simulink model "Offline_MiL_Sim_Public"  (R2024a)
settings: Solver=ode1  StartTime=0.0  StopTime=inf  FixedStep=step_size  RelTol=1e-3  EnableMultiTasking=on
PostLoadFcn:
  | if any(exist('dsrtsu_mdlpostloadfcn', 'file') ~= 0), dsrtsu_mdlpostloadfcn('Execute', bdroot); end
InitFcn:
  | , if any(exist('rtifpga_mdlclblib', 'file') ~= 0), rtifpga_mdlclblib('Init', bdroot); end,
  | , if any(exist('dsmpb_private', 'file') ~= 0), dsmpb_private('dsmpb_mdlclblib', 'Init', bdroot); end,
undefined symbols (not defined in the file or in its folder): Af, break_criteria, C_r, C_w, Cd, CurrentLosses, dens, DiscIntNeverNeededParam, FDR, fr, Friction, gain_Twr, grade_track, grav, IronLosses, Kp_c, lbh_ac, lbx_ac, lbx_ac_e, lbx_mhe, M_EM_acc_0, M_EM_acc_max, M_EM_brk_min, M_gen_max, M_mot_max, mpc_init_EM_acc, mpc_init_EM_brk, mpc_init_fric_brk, mps_kmh, Mv, n_0, n_em_max, n_gen_max, n_mot_max, n_vec, nout, numHiddenUnits, options, options_mhe, optparam, P, parameter_0, Q, R, r_dyn, R_w_c, R_w_e, R_w_r, rps_rpm, s_track, SE_selector_sim, start_distance_check, step_size, T_c, T_cool, T_e, T_init, T_max, t_mpc_on, T_r_0 ... (+21)
libraries: simulink x3, matrix_library x2, deeplib x1
(part 1 of 2)
PreSaveFcn:
  | if any(exist('dsmpb_private', 'file') ~= 0), dsmpb_private('dsmpb_mdlclblib', 'PreSave', bdroot); end
CloseFcn:
  | if any(exist('dsmpb_private', 'file') ~= 0), dsmpb_private('dsmpb_mdlclblib', 'Close', bdroot); end
settings Model: FPTRunName=Active  DSMPB_ID_DATA={}  RTICANMMDATA=struct('GeneralSetupData',struct('modelroot','D:\Git_Winkler\nmpc_wang','generalsettings',struct('filesettings',struct('destfolder',struct('Name','RTICANMM_FILES','Check',1),'buildfolder',struct('Name','.','Check',1),'AbsDestfolder',struct('Name','D:\Git_Winkler\nmpc_wang\RTICANMM_FILES'),'AbsBuildfolder',struct('Name','D:\Git_Winkler\nmpc_wang'))),'options',struct('addpaths',1,'rmpaths',1,'addtrcexclusion',true,'cannavigator',struct('checkmonitoring',0),'show_usrtrc',0,'use_usrtrc',0),'advanced',struct('options',ones(1,100)),'MPSetup',{{}},'RTI',struct('Type','DSRT','Ver','4.6','Date','02-Nov-2021'),'modelname','mpc_ww_Scalexio_Offline_LSTM_v3_2021a','block','mpc_ww_Scalexio_Offline_LSTM_v3_2021a'))  DSRTSU_INTERNAL_RTIFPGA=170  DSRTSU_INTERNAL_RTISTBM_VER=1.4.3  NumberOfSteps=10  PacingRate=1.600000  Creator=The MathWorks, Inc.  LastModifiedBy=winkler_a
settings SolverCC: AlgebraicLoopSolver=LineSearch  AutoInsertRateTranBlk=on
settings DataIOCC: SaveFormat=Array  SignalLogging=off  DSMLogging=off  ReturnWorkspaceOutputs=off  SignalLoggingName=sigsOut
settings OptimizationCC: BlockReduction=off  BooleanDataType=off  ConditionallyExecuteInputs=off  DefaultParameterBehavior=Inlined  OptimizeBlockIOStorage=off  BufferReuse=off  ReuseModelBlockBuffer=off  GlobalBufferReuse=off  ExpressionFolding=off  ExpressionDepthLimit=2147483647  LocalBlockOutputs=off  InitFltsAndDblsToZero=on  OptimizeDataStoreBuffers=off  BusAssignmentInplaceUpdate=off
settings DebuggingCC: SaveWithParameterizedLinksMsg=none  MultiTaskDSMMsg=warning  MultiTaskCondExecSysMsg=none  TasksWithSamePriorityMsg=none  FcnCallInpInsideContextMsg=warning  UnconnectedLineMsg=warning  StateNameClashWarn=warning  SFUnexpectedBacktrackingDiag=warning  SFNoUnconditionalDefaultTransitionDiag=warning  ArithmeticOperatorsInVariantConditions=warning
settings HardwareCC: ProdBitPerPointer=32  ProdBitPerSizeT=32  ProdBitPerPtrDiffT=32  ProdLargestAtomicInteger=Integer  ProdWordSize=32  ProdHWDeviceType=Custom Processor->Custom  TargetBitPerPointer=64  TargetBitPerSizeT=64  TargetBitPerPtrDiffT=64  TargetLongLongMode=on  TargetIntDivRoundTo=Zero  TargetEndianess=LittleEndian  TargetWordSize=64  TargetHWDeviceType=MATLAB Host
settings ModelReferenceCC: EnableRefExpFcnMdlSchedulingChecks=on  PropagateSignalLabelsOutOfModel=off
settings SFSimCC: SimUseLocalCustomCode=off  MATLABDynamicMemAlloc=off  CustomCodeUndefinedFunction=UseInterfaceOnly
settings RTWCC: Description=dSPACE Run-Time Target (for VEOS and ConfigurationDesk)  SystemTargetFile=dsrt.tlc  GenCodeOnly=on  MakeCommand=make_dsrt  TemplateMakefile=dsrt_default_tmf  RTWVerbose=off  RTWUseLocalCustomCode=off  GPUComputeCapability=3.5  DLArmComputeVersion=19.05
settings CodeAppCC: StateflowObjectComments=on
settings STFCustomTargetCC: TargetLangStandard=C89/C90 (ANSI)  ParMdlRefBuildCompliant=on  GRTInterface=off  UseToolchainInfoCompliant=off  SystemTargetFile=dsrt.tlc
settings GRTTargetCC: TargetLangStandard=C89/C90 (ANSI)  CompOptLevelCompliant=off  ConcurrentExecutionCompliant=off  CombineOutputUpdateFcns=off  MatFileLogging=off  CPPClassGenCompliant=off  UseToolchainInfoCompliant=off
settings ConfigComp: CovMetricSettings=dw  CovSaveCumulativeToWorkspaceVar=on  CovSaveSingleToWorkspaceVar=on  CovExternalEMLEnable=off  CovSFcnEnable=off

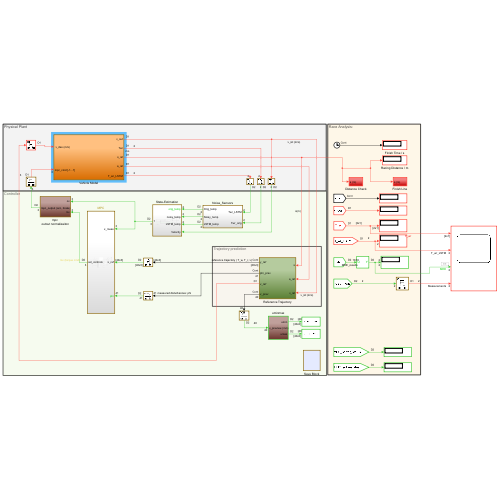
[thumbnail: Simulink's stored preview of the top-level diagram]
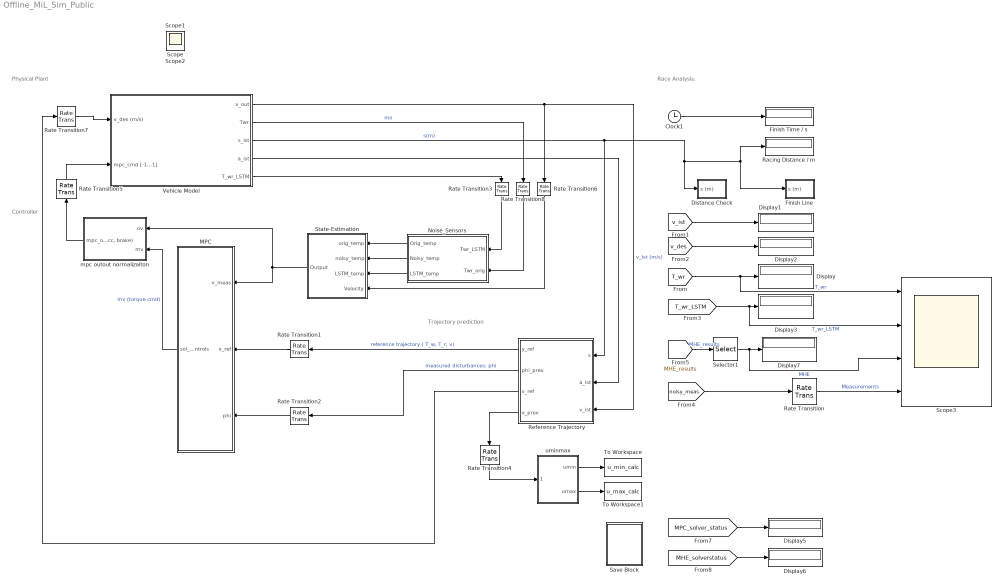
== system Offline_MiL_Sim_Public ==
  note: Trajectory prediction
  note: Controller
  note: Physical Plant
  note: Race Analysis:
  Clock1 : Clock
  Display{,1..3,5..7} (7 alike) : Display
  Distance Check : Subsystem
  Finish Line : Subsystem
  Finish Time / s : Display
  MPC : Subsystem
  Noise_Sensors : Subsystem
  Racing Distance / m : Display
  Rate Transition : RateTransition
  Rate Transition1 : RateTransition  InitialCondition=X0_ref  OutPortSampleTime=options.Ts
  Rate Transition2 : RateTransition  InitialCondition=parameter_0(1:(options.P+1))  OutPortSampleTime=options.Ts
  Rate Transition3 : RateTransition  Deterministic=off  InitialCondition=[T_w_0, T_r_0]  OutPortSampleTime=options.Ts
  Rate Transition4 : RateTransition  InitialCondition=v_0  OutPortSampleTime=options.Ts
  Rate Transition5 : RateTransition  InitialCondition=[mpc_init_EM_acc, mpc_init_EM_brk, mpc_init_fric_brk]  OutPortSampleTime=step_size
  Rate Transition6 : RateTransition  Deterministic=off  InitialCondition=[v_0]  OutPortSampleTime=options.Ts
  Rate Transition7 : RateTransition  InitialCondition=v_0  OutPortSampleTime=step_size
  Rate Transition8 : RateTransition  Deterministic=off  InitialCondition=[T_w_0, T_r_0]  OutPortSampleTime=options.Ts
  Reference Trajectory : Subsystem
  Save Block : Subsystem
  Scope3 : Scope  NumInputPorts=4
  Selector1 : Selector  InputPortWidth=18  IndexOptions=Index vector (dialog)  Indices=[1:2]  OutputSizes=1
  State-Estimation : Subsystem
  To Workspace : ToWorkspace  VariableName=u_min_calc  SaveFormat=Timeseries  SampleTime=-1
  To Workspace1 : ToWorkspace  VariableName=u_max_calc  SaveFormat=Timeseries  SampleTime=-1
  Vehicle Model : Subsystem
  mpc outout normalizaiton : Subsystem
  uminmax : Subsystem
  Scope : Scope
  Scope1 : Scope
  Scope2 : Scope
  wires:
  Reference Trajectory/2(phi_prev) -> Rate Transition2/1  "measured disturbances: phi"
  Vehicle Model/3(s_ist) -> Reference Trajectory/1(s), Racing Distance / m/1, Finish Line/1(s (m)), Distance Check/1(s (m))  "s(m)"
  MPC/1(sol_controls) -> mpc outout normalizaiton/2(mv)  "mv (torque cmd)"
  Vehicle Model/1(v_out) -> Rate Transition6/1, Reference Trajectory/3(v_ist)  "v_ist (m/s)"
  mpc outout normalizaiton/1("mpc_output (acc, brake)") -> Rate Transition5/1
  Reference Trajectory/1(y_ref) -> Rate Transition1/1  "reference trajectory ( T_w, T_r, v)"
  Vehicle Model/4(a_ist) -> Reference Trajectory/2(a_ist)
  Clock1/1 -> Finish Time / s/1
  Rate Transition2/1 -> MPC/3(phi)
  Rate Transition1/1 -> MPC/2(x_ref)
  Rate Transition5/1 -> Vehicle Model/2(mpc_cmd [-1...1])
  Rate Transition4/1 -> uminmax/1(v_preview (m/s))
  Reference Trajectory/3(v_ref) -> Rate Transition7/1
  Rate Transition7/1 -> Vehicle Model/1(" v_des (m/s)")
  Reference Trajectory/4(v_prev) -> Rate Transition4/1
  uminmax/1(umin) -> To Workspace/1
  uminmax/2(umax) -> To Workspace1/1
  [T_wr] -> Scope3/1, Display/1  "T_wr"
  [v_ist] -> Display1/1
  [v_des] -> Display2/1
  [T_wr_LSTM] -> Scope3/2, Display3/1  "T_wr_LSTM"
  State-Estimation/1(Output) -> mpc outout normalizaiton/1(ov), MPC/1(x_meas)
  Noise_Sensors/1(Orig_temp) -> State-Estimation/1(orig_temp)
  [MHE_results] -> Selector1/1  "MHE_results"
  Vehicle Model/5(T_wr_LSTM) -> Rate Transition3/1
  Selector1/1 -> Scope3/3, Display7/1  "MHE"
  Noise_Sensors/2(Noisy_temp) -> State-Estimation/2(noisy_temp)
  [noisy_meas] -> Rate Transition/1
  Rate Transition/1 -> Scope3/4  "Measurements"
  Rate Transition6/1 -> State-Estimation/4(Velocity)
  Vehicle Model/2(Twr) -> Rate Transition8/1  "mo"
  Rate Transition8/1 -> Noise_Sensors/2(Twr_orig)
  Rate Transition3/1 -> Noise_Sensors/1(Twr_LSTM)
  Noise_Sensors/3(LSTM_temp) -> State-Estimation/3(LSTM_temp)
  [MPC_solver_status] -> Display5/1
  [MHE_solverstatus] -> Display6/1

== system Offline_MiL_Sim_Public/Distance Check ==
  s (m) : Inport
  Distance Change Security Check : Subsystem
  Stop Simulation : Stop
  To Workspace24 : ToWorkspace  VariableName=bool_stop  SampleTime=-1
      settings: MaxDataPoints=1  Save2DSignal=2-D array (concatenate along first dimension)
  wires:
  s (m)/1 -> Distance Change Security Check/1(s)
  Distance Change Security Check/1(bool_stop) -> Stop Simulation/1, To Workspace24/1

== system Offline_MiL_Sim_Public/Finish Line ==
  s (m) : Inport
  Constant : Constant  Value=0
  Constant1 : Constant
  Stop Simulation : Stop
  s>finish line : Switch  Threshold=s_track(end)  SaturateOnIntegerOverflow=off  InputSameDT=off
  s_ist : Gain
  wires:
  s (m)/1 -> s_ist/1
  Constant1/1 -> s>finish line/1
  Constant/1 -> s>finish line/3
  s>finish line/1 -> Stop Simulation/1
  s_ist/1 -> s>finish line/2

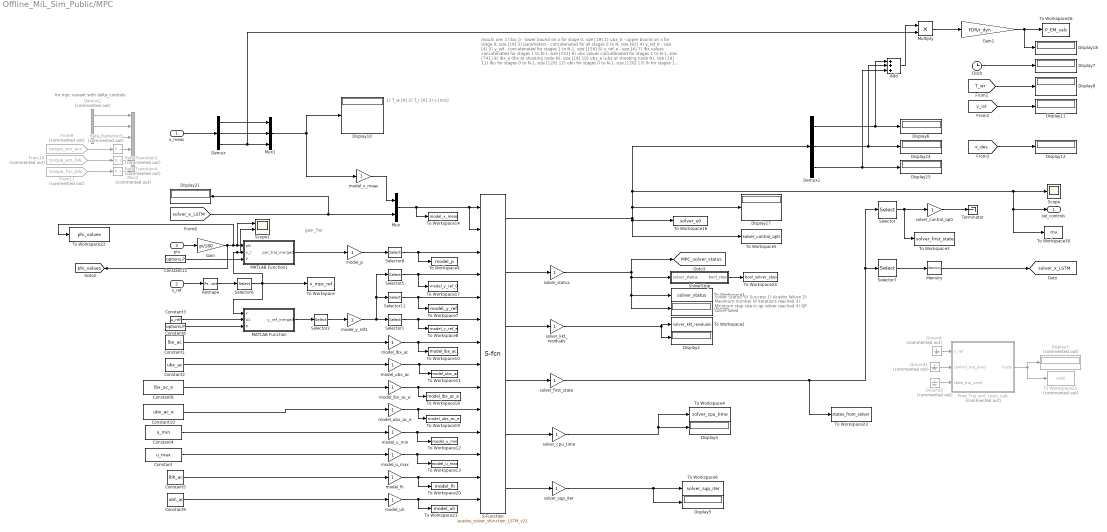
== system Offline_MiL_Sim_Public/MPC ==
  note: for mpc variant with delta_controls
  note: gain_Twr
  note: Inputs are:
      | 1) lbx_0 - lower bound on x for stage 0, size [19]
      | 2) ubx_0 - upper bound on x for stage 0, size [19]
      | 3) parameters - concatenated for all stages 0 to N, size [82]
      | 4) y_ref_0 - size [4]
      | 5) y_ref - concatenated for stages 1 to N-1, size [156]
      | 6) y_ref_e - size [4]
      | 7) lbx values concatenated for stages 1 to N-1, size [741]
      | 8) ubx values concatenated for stages 1 to N-1, size [741]
      | 9) lbx_e (lbx at shooting node N), size [19]
      | 10) ubx_e (ubx at shooting node N), size [19]
      | 11) lbu for stages 0 to N-1, size [120]
      | 12) ubu for stages 0 to N-1, size [120]
      | 13) lh for stages 1 to N-1, size [156]
      | 14) uh for stages 1 to N-1, size [156]
      | 15) cost_W in column-major format, that is set for all intermediate stages: 1 to N-1, size [16]
      |
      | Outputs are:
      | 1) u0, control input at node 0, size [3]
      | 2) acados solver status (0 = SUCCESS)
      | 3) KKT residual
      | 4) x1, state at node 1
      | 5) CPU time
      | 6) SQP iterations
  note: Solver Status:
      | 0) Success
      | 1) Acados failure
      | 2) Maximum number of iterations reached
      | 3) Minimum step size in qp solver reached
      | 4) QP solver failed
  note: 1) T_w [K]
      | 2) T_r [K]
      | 3) v [m/s]
  x_meas : Inport
  x_ref : Inport  Port=2
  phi : Inport  Port=3
  Add : Sum  Inputs=+++
  Clock : Clock
  Constant : Constant  Value=u_max  SampleTime=options.Ts
  Constant1 : Constant  Value=lbx_ac  SampleTime=options.Ts
  Constant10 : Constant  Value=ubx_ac_e  SampleTime=options.Ts
  Constant11 : Constant  Value=options.P  SampleTime=options.Ts
  Constant2 : Constant  Value=ubx_ac  SampleTime=options.Ts
  Constant3 : Constant  Value=u_ref  SampleTime=options.Ts
  Constant4 : Constant  Value=u_min  VectorParams1D=off  SampleTime=options.Ts
  Constant5 : Constant  Value=lbh_ac  SampleTime=options.Ts
  Constant6 : Constant  Value=options.P  SampleTime=options.Ts
  Constant8 : Constant  Value=lbx_ac_e  SampleTime=options.Ts
  Constant9 : Constant  Value=ubh_ac  SampleTime=options.Ts
  Demux : Demux  Outputs=3
  Demux1 : Demux  Outputs=options.n_controls
  Demux2 : Demux  Commented=on  Outputs=3
  Display{,2,4..8,10..12,17..18,21,24..25} (15 alike) : Display
  Display3 : Display  Commented=on
  From10 : From  Commented=on  GotoTag=torque_em_brk  TagVisibility=global
  From11 : From  Commented=on  GotoTag=torque_fric_brk  TagVisibility=global
  From9 : From  Commented=on  GotoTag=torque_em_acc  TagVisibility=global
  Gain : Gain  Gain=pi/180
  Gain1 : Gain  Gain=FDR/r_dyn
  Ground : Ground  Commented=on
  Ground1 : Ground  Commented=on
  Ground2 : Ground  Commented=on
  MATLAB Function : MATLAB Function  TreatAsAtomicUnit=on
  MATLAB Function1 : MATLAB Function  TreatAsAtomicUnit=on
  Memory : Memory  InheritSampleTime=on
  Multiply : Product
  Mux : Mux  Inputs=2
  Mux1 : Mux  Inputs=3
  Mux2 : Mux  Commented=on  Inputs=6
  Pred_Traj_and_costs_calc : Subsystem  Commented=on
  Rate Transition3 : RateTransition  Commented=on  InitialCondition=M_EM_acc_0  OutPortSampleTime=options.Ts
  Rate Transition4 : RateTransition  Commented=on  InitialCondition=M_EM_acc_0  OutPortSampleTime=options.Ts
  Rate Transition5 : RateTransition  Commented=on  InitialCondition=M_EM_acc_0  OutPortSampleTime=options.Ts
  Reshape : Reshape
  S-Function : S-Function  FunctionName=acados_solver_sfunction_LSTM_v21  SFunctionDeploymentMode=off  EnableBusSupport=off
  Scope : Scope
  Scope1 : Scope  NumInputPorts=2
  Selector : Selector  InputPortWidth=options.n_states  IndexOptions=Index vector (dialog)  Indices=[options.n_states-2:options.n_states]  OutputSizes=1
  Selector1 : Selector  IndexOptions=Index vector (dialog)  Indices=[((options.P-1)*options.n_outputs+1):(options.P*(options.n_outputs))]  OutputSizes=1
  Selector11 : Selector  IndexOptions=Index vector (dialog)  Indices=[1:((options.P-1)*(options.n_outputs))]  OutputSizes=1
  Selector2 : Selector  InputPortWidth=160  IndexOptions=Index vector (dialog)  Indices=[1:(options.P*(options.n_outputs))]  OutputSizes=1
  Selector5 : Selector  IndexOptions=Index vector (dialog)  Indices=[1:(options.n_outputs)]  OutputSizes=1
  Selector6 : Selector  InputPortWidth=options.P*(3)  IndexOptions=Index vector (dialog)  Indices=[(options. P*2+1):(options.P*3)]  OutputSizes=1
  Selector7 : Selector  InputPortWidth=options.n_states  IndexOptions=Index vector (dialog)  Indices=[options.n_states_bound+1:options.n_states]  OutputSizes=1
  Selector8 : Selector  InputPortWidth=160  IndexOptions=Index vector (dialog)  Indices=[1:((options.P+1)*(options.n_parameter))]  OutputSizes=1
  SolverStop : Subsystem
  Terminator : Terminator
  To Workspace : ToWorkspace  VariableName=v_mpc_ref  SampleTime=-1
  To Workspace1 : ToWorkspace  VariableName=solver_status  SampleTime=options.Ts
      settings: Save2DSignal=2-D array (concatenate along first dimension)
  To Workspace10 : ToWorkspace  VariableName=model_lbx_ac  SampleTime=-1
  To Workspace11 : ToWorkspace  VariableName=model_ubx_ac  SampleTime=-1
  To Workspace12 : ToWorkspace  VariableName=model_u_min  SampleTime=-1
  To Workspace13 : ToWorkspace  VariableName=model_u_max  SampleTime=-1
  To Workspace14 : ToWorkspace  VariableName=model_x_meas  SampleTime=-1
  To Workspace16 : ToWorkspace  VariableName=solver_u0  SampleTime=-1
      settings: MaxDataPoints=1  Save2DSignal=2-D array (concatenate along first dimension)
  To Workspace17 : ToWorkspace  VariableName=model_y_ref_0  SampleTime=-1
  To Workspace18 : ToWorkspace  VariableName=model_lbx_ac_e  SampleTime=-1
  To Workspace19 : ToWorkspace  VariableName=model_ubx_ac_e  SampleTime=-1
  To Workspace2 : ToWorkspace  VariableName=solver_kkt_residuals  SampleTime=options.Ts
      settings: Save2DSignal=2-D array (concatenate along first dimension)
  To Workspace20 : ToWorkspace  VariableName=model_lh  SampleTime=-1
  To Workspace21 : ToWorkspace  VariableName=model_uh  SampleTime=-1
  To Workspace22 : ToWorkspace  VariableName=phi_values  SampleTime=-1
  To Workspace23 : ToWorkspace  VariableName=states_from_solver  SampleTime=-1
      settings: Save2DSignal=2-D array (concatenate along first dimension)
  To Workspace24 : ToWorkspace  VariableName=bool_solver_stop  SampleTime=-1
      settings: MaxDataPoints=1  Save2DSignal=2-D array (concatenate along first dimension)
  To Workspace25 : ToWorkspace  Commented=on  VariableName=cost  SampleTime=-1
  To Workspace26 : ToWorkspace  VariableName=P_EM_calc  SampleTime=-1
      settings: Save2DSignal=2-D array (concatenate along first dimension)
  To Workspace3 : ToWorkspace  VariableName=solver_first_state  SampleTime=options.Ts
      settings: Save2DSignal=2-D array (concatenate along first dimension)
  To Workspace30 : ToWorkspace  VariableName=mv  SampleTime=-1
  To Workspace4 : ToWorkspace  VariableName=solver_cpu_time  SampleTime=options.Ts
      settings: Save2DSignal=2-D array (concatenate along first dimension)
  To Workspace5 : ToWorkspace  VariableName=solver_control_opti  SampleTime=options.Ts
      settings: Save2DSignal=2-D array (concatenate along first dimension)
  To Workspace6 : ToWorkspace  VariableName=solver_sqp_iter  SampleTime=options.Ts
      settings: Save2DSignal=2-D array (concatenate along first dimension)
  To Workspace7 : ToWorkspace  VariableName=model_y_ref  SampleTime=-1
  To Workspace8 : ToWorkspace  VariableName=model_y_ref_e  SampleTime=-1
  To Workspace9 : ToWorkspace  VariableName=model_p  SampleTime=-1
  model_lbx_ac : Gain
  model_lbx_ac_e : Gain
  model_lh : Gain
  model_p : Gain
  model_u_max : Gain
  model_u_min : Gain
  model_ubx_ac : Gain
  model_ubx_ac_e : Gain
  model_uh : Gain
  model_x_meas : Gain
  model_y_ref1 : Gain
  solver_control_opti : Gain
  solver_cpu_time : Gain
  solver_first_state : Gain
  solver_kkt_residuals : Gain
  solver_sqp_iter : Gain
  solver_status : Gain
  sol_controls : Outport  VectorParamsAs1DForOutWhenUnconnected=off
  tag scope: MPC_solver_status=global, phi_values=global, solver_x_LSTM=global
  wires:
  phi/1 -> Gain/1
  solver_kkt_residuals/1 -> Display2/1, To Workspace2/1
  solver_cpu_time/1 -> To Workspace4/1, Display4/1
  solver_sqp_iter/1 -> Display5/1, To Workspace6/1
  Selector11/1 -> To Workspace7/1, S-Function/5
  model_p/1 -> Selector8/1
  model_lbx_ac/1 -> S-Function/7, To Workspace10/1
  model_ubx_ac/1 -> S-Function/8, To Workspace11/1
  model_u_min/1 -> To Workspace12/1, S-Function/11
  model_u_max/1 -> S-Function/12, To Workspace13/1
  Selector6/1 -> To Workspace/1, Scope1/2, MATLAB Function1/2(v_r), MATLAB Function/1(x)
  Reshape/1 -> Selector6/1
  Constant3/1 -> MATLAB Function/2(u1)
  SolverStop/1(bool_stop) -> To Workspace24/1
  Clock/1 -> Display7/1
  [v_ist] -> Display11/1
  [v_des] -> Display12/1
  [T_wr] -> Display8/1
  solver_status/1 -> [MPC_solver_status], Display/1, To Workspace1/1, SolverStop/1(solver_status)
  x_meas/1 -> Demux/1
  Demux/2 -> Mux1/2
  Demux/1 -> Mux1/1
  Selector1/1 -> S-Function/6, To Workspace8/1
  Gain/1 -> [phi_values], To Workspace22/1, Scope1/1, MATLAB Function1/1(phi)
  Gain1/1 -> Display18/1, To Workspace26/1
  Multiply/1 -> Gain1/1
  Demux/3 -> Mux1/3, Multiply/2
  Constant4/1 -> model_u_min/1
  Constant/1 -> model_u_max/1
  MATLAB Function/1(y_ref_merged) -> Selector2/1
  Selector2/1 -> model_y_ref1/1
  x_ref/1 -> Reshape/1
  Pred_Traj_and_costs_calc/1(Costs) -> Display3/1, To Workspace25/1
  Constant6/1 -> MATLAB Function/3(P)
  Add/1 -> Multiply/1
  Ground/1 -> Pred_Traj_and_costs_calc/1(v_ref)
  Ground2/1 -> Pred_Traj_and_costs_calc/3(state_traj_pred)
  Ground1/1 -> Pred_Traj_and_costs_calc/2(control_traj_pred)
  S-Function/1 -> Display17/1, Scope/1, sol_controls/1, To Workspace30/1, Demux1/1, To Workspace5/1, To Workspace16/1
  solver_first_state/1 -> To Workspace23/1, Selector/1, Selector7/1
  Selector5/1 -> S-Function/4, To Workspace17/1
  Constant1/1 -> model_lbx_ac/1
  Constant2/1 -> model_ubx_ac/1
  Constant5/1 -> model_lh/1
  Constant9/1 -> model_uh/1
  model_lh/1 -> S-Function/13, To Workspace20/1
  model_uh/1 -> S-Function/14, To Workspace21/1
  model_y_ref1/1 -> Selector11/1, Selector5/1, Selector1/1
  Constant8/1 -> model_lbx_ac_e/1
  Constant10/1 -> model_ubx_ac_e/1
  model_lbx_ac_e/1 -> S-Function/9, To Workspace18/1
  model_ubx_ac_e/1 -> S-Function/10, To Workspace19/1
  Selector/1 -> To Workspace3/1, solver_control_opti/1
  Mux/1 -> To Workspace14/1, S-Function/2, S-Function/1
  Selector7/1 -> Memory/1
  [solver_x_LSTM] -> Display21/1, Mux/2
  model_x_meas/1 -> Mux/1
  solver_control_opti/1 -> Terminator/1
  From9/1 -> Rate Transition5/1
  From11/1 -> Rate Transition4/1
  From10/1 -> Rate Transition3/1
  Rate Transition4/1 -> Mux2/6
  Demux2/2 -> Mux2/2
  Demux2/1 -> Mux2/1
  Rate Transition3/1 -> Mux2/5
  Rate Transition5/1 -> Mux2/4
  Demux2/3 -> Mux2/3
  Memory/1 -> [solver_x_LSTM]
  Demux1/1 -> Add/1, Display6/1
  Demux1/2 -> Add/2, Display24/1
  Demux1/3 -> Display25/1, Add/3
  Mux1/1 -> Display10/1, model_x_meas/1
  Constant11/1 -> MATLAB Function1/3(P)
  MATLAB Function1/1(par_traj_merged) -> model_p/1
  Selector8/1 -> S-Function/3, To Workspace9/1
  S-Function/6 -> solver_sqp_iter/1
  S-Function/2 -> solver_status/1
  S-Function/3 -> solver_kkt_residuals/1
  S-Function/5 -> solver_cpu_time/1
  S-Function/4 -> solver_first_state/1

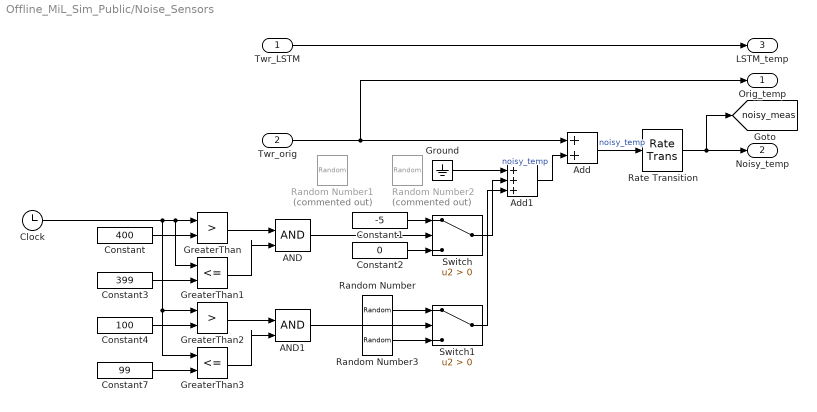
== system Offline_MiL_Sim_Public/Noise_Sensors ==
  Twr_LSTM : Inport
  Twr_orig : Inport  Port=2
  AND : Logic  IconShape=distinctive  AllPortsSameDT=off  OutDataTypeStr=boolean
  AND1 : Logic  IconShape=distinctive  AllPortsSameDT=off  OutDataTypeStr=boolean
  Add : Sum
  Add1 : Sum  Inputs=+++
  Clock : Clock
  Constant : Constant  Value=400
  Constant1 : Constant  Value=-5
  Constant2 : Constant  Value=0
  Constant3 : Constant  Value=399
  Constant4 : Constant  Value=100
  Constant7 : Constant  Value=99
  GreaterThan : RelationalOperator  Operator=>  OutDataTypeStr=boolean  RndMeth=Simplest  InputSameDT=off
  GreaterThan1 : RelationalOperator  Operator=<=  OutDataTypeStr=boolean  RndMeth=Simplest  InputSameDT=off
  GreaterThan2 : RelationalOperator  Operator=>  OutDataTypeStr=boolean  RndMeth=Simplest  InputSameDT=off
  GreaterThan3 : RelationalOperator  Operator=<=  OutDataTypeStr=boolean  RndMeth=Simplest  InputSameDT=off
  Ground : Ground
  Random Number : RandomNumber  Variance=3  SampleTime=0.1
  Random Number1 : RandomNumber  Commented=on  Mean=-2  Variance=0.5  SampleTime=0.5
  Random Number2 : RandomNumber  Commented=on  Variance=0.1  SampleTime=0.1
  Random Number3 : RandomNumber  Mean=-2  Variance=0.1  SampleTime=0.1
  Rate Transition : RateTransition
  Switch : Switch  Criteria=u2 > Threshold  SaturateOnIntegerOverflow=off  InputSameDT=off
  Switch1 : Switch  Criteria=u2 > Threshold  SaturateOnIntegerOverflow=off  InputSameDT=off
  Orig_temp : Outport
  Noisy_temp : Outport  Port=2
  LSTM_temp : Outport  Port=3
  tag scope: noisy_meas=global
  wires:
  Add/1 -> Rate Transition/1  "noisy_temp"
  Twr_LSTM/1 -> LSTM_temp/1
  Twr_orig/1 -> Orig_temp/1, Add/1
  Clock/1 -> GreaterThan3/1, GreaterThan2/1, GreaterThan1/1, GreaterThan/1
  Constant/1 -> GreaterThan/2
  Constant1/1 -> Switch/1
  Constant2/1 -> Switch/3
  Add1/1 -> Add/2  "noisy_temp"
  Switch/1 -> Add1/2
  Ground/1 -> Add1/1
  Rate Transition/1 -> [noisy_meas], Noisy_temp/1
  Constant3/1 -> GreaterThan1/2
  AND/1 -> Switch/2
  GreaterThan1/1 -> AND/2
  GreaterThan/1 -> AND/1
  GreaterThan2/1 -> AND1/1
  GreaterThan3/1 -> AND1/2
  AND1/1 -> Switch1/2
  Constant7/1 -> GreaterThan3/2
  Random Number/1 -> Switch1/1
  Constant4/1 -> GreaterThan2/2
  Switch1/1 -> Add1/3
  Random Number3/1 -> Switch1/3

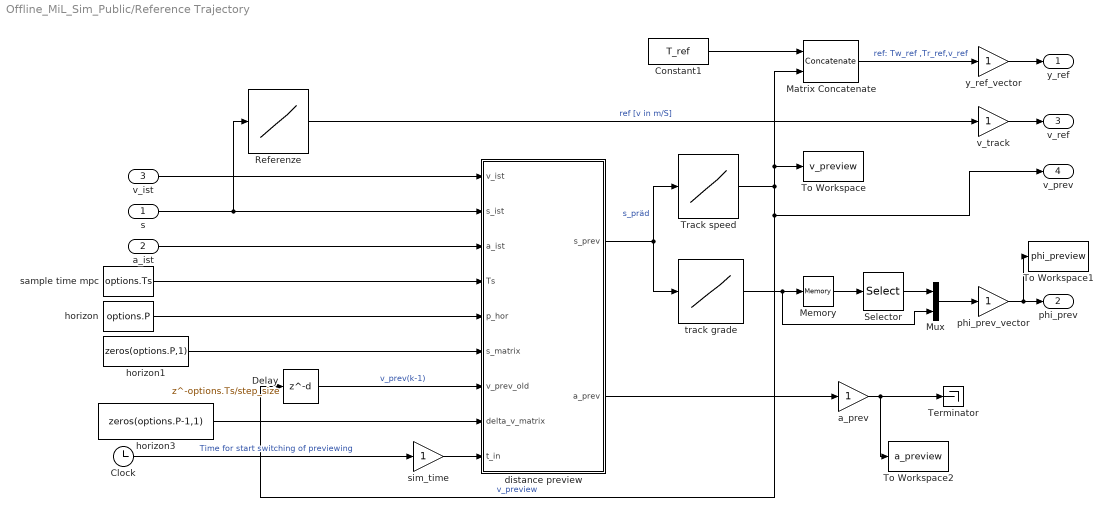
== system Offline_MiL_Sim_Public/Reference Trajectory ==
  s : Inport  PortDimensions=1
  a_ist : Inport  Port=2  PortDimensions=1
  v_ist : Inport  Port=3  PortDimensions=1
  Clock : Clock
  Constant1 : Constant  Value=T_ref
  Delay : Delay  DelayLength=options.Ts/step_size  InitialCondition=0
  Matrix Concatenate : Concatenate  Mode=Multidimensional array  ConcatenateDimension=2
  Memory : Memory  InitialCondition=grade_track(1:options.P)
  Mux : Mux  Inputs=2
  Referenze : Lookup_n-D  NumberOfTableDimensions=1  BreakpointsForDimension1=s_track  Table=v_track  InternalRulePriority=Speed  RndMeth=Simplest
  Selector : Selector  InputPortWidth=options.P  IndexOptions=Index vector (dialog)  Indices=[1]  OutputSizes=1
  Terminator : Terminator
  To Workspace : ToWorkspace  VariableName=v_preview  SampleTime=-1
      settings: MaxDataPoints=1  Save2DSignal=2-D array (concatenate along first dimension)
  To Workspace1 : ToWorkspace  VariableName=phi_preview  SampleTime=-1
      settings: MaxDataPoints=1  Save2DSignal=2-D array (concatenate along first dimension)
  To Workspace2 : ToWorkspace  VariableName=a_preview  SampleTime=-1
      settings: MaxDataPoints=1  Save2DSignal=2-D array (concatenate along first dimension)
  "Track speed " : Lookup_n-D  NumberOfTableDimensions=1  BreakpointsForDimension1=s_track  Table=v_track  InternalRulePriority=Speed  RndMeth=Simplest
  a_prev : Gain
  distance preview : MATLAB Function  TreatAsAtomicUnit=on
  horizon : Constant  Value=options.P
  horizon1 : Constant  Value=zeros(options.P,1)
  horizon3 : Constant  Value=zeros(options.P-1,1)
  phi_prev_vector : Gain
  sample time mpc : Constant  Value=options.Ts  VectorParams1D=off
  sim_time : Gain
  track grade : Lookup_n-D  NumberOfTableDimensions=1  BreakpointsForDimension1=s_track  Table=grade_track  InternalRulePriority=Speed  RndMeth=Simplest
  v_track : Gain
  y_ref_vector : Gain
  y_ref : Outport  VectorParamsAs1DForOutWhenUnconnected=off
  phi_prev : Outport  Port=2  VectorParamsAs1DForOutWhenUnconnected=off
  v_ref : Outport  Port=3  VectorParamsAs1DForOutWhenUnconnected=off
  v_prev : Outport  Port=4  VectorParamsAs1DForOutWhenUnconnected=off
  wires:
  s/1 -> Referenze/1, distance preview/2(s_ist)
  Matrix Concatenate/1 -> y_ref_vector/1  "ref: Tw_ref ,Tr_ref,v_ref"
  Referenze/1 -> v_track/1  "ref [v in m/S]"
  sample time mpc/1 -> distance preview/4(Ts)
  distance preview/1(s_prev) -> track grade/1, "Track speed "/1  "s_präd"
  "Track speed "/1 -> v_prev/1, Delay/1, To Workspace/1, Matrix Concatenate/2  "v_preview"
  a_ist/1 -> distance preview/3(a_ist)
  v_ist/1 -> distance preview/1(v_ist)
  horizon/1 -> distance preview/5(p_hor)
  horizon1/1 -> distance preview/6(s_matrix)
  Delay/1 -> distance preview/7(v_prev_old)  "v_prev(k-1)"
  horizon3/1 -> distance preview/8(delta_v_matrix)
  Clock/1 -> sim_time/1  "Time for start switching of previewing"
  Constant1/1 -> Matrix Concatenate/1
  sim_time/1 -> distance preview/9(t_in)
  distance preview/2(a_prev) -> a_prev/1
  a_prev/1 -> To Workspace2/1, Terminator/1
  v_track/1 -> v_ref/1
  y_ref_vector/1 -> y_ref/1
  Memory/1 -> Selector/1
  Selector/1 -> Mux/1
  track grade/1 -> Mux/2, Memory/1
  Mux/1 -> phi_prev_vector/1
  phi_prev_vector/1 -> To Workspace1/1, phi_prev/1

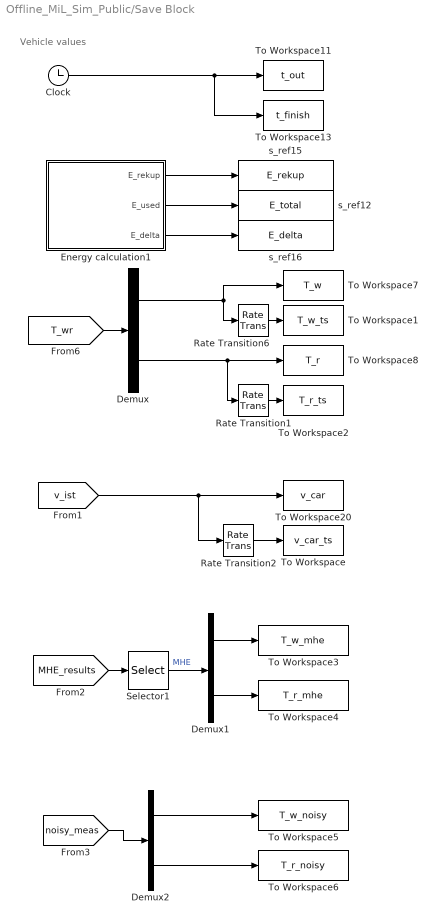
== system Offline_MiL_Sim_Public/Save Block ==
  note: Vehicle values
  Clock : Clock
  Demux : Demux  Outputs=2
  Demux1 : Demux  Outputs=2
  Demux2 : Demux  Outputs=2
  Energy calculation1 : Subsystem
  Rate Transition1 : RateTransition  InitialCondition=T_r_0  OutPortSampleTime=options.Ts
  Rate Transition2 : RateTransition  OutPortSampleTime=options.Ts
  Rate Transition6 : RateTransition  InitialCondition=T_w_0  OutPortSampleTime=options.Ts
  Selector1 : Selector  InputPortWidth=18  IndexOptions=Index vector (dialog)  Indices=[1:2]  OutputSizes=1
  To Workspace : ToWorkspace  VariableName=v_car_ts  SampleTime=-1
      settings: Save2DSignal=2-D array (concatenate along first dimension)
  To Workspace1 : ToWorkspace  VariableName=T_w_ts  SampleTime=-1
      settings: Save2DSignal=2-D array (concatenate along first dimension)
  To Workspace11 : ToWorkspace  VariableName=t_out  SampleTime=-1
      settings: Save2DSignal=2-D array (concatenate along first dimension)
  To Workspace13 : ToWorkspace  VariableName=t_finish  SampleTime=-1
      settings: MaxDataPoints=1  Save2DSignal=2-D array (concatenate along first dimension)
  To Workspace2 : ToWorkspace  VariableName=T_r_ts  SampleTime=-1
      settings: Save2DSignal=2-D array (concatenate along first dimension)
  To Workspace20 : ToWorkspace  VariableName=v_car  SampleTime=-1
      settings: Save2DSignal=2-D array (concatenate along first dimension)
  To Workspace3 : ToWorkspace  VariableName=T_w_mhe  SampleTime=-1
      settings: Save2DSignal=2-D array (concatenate along first dimension)
  To Workspace4 : ToWorkspace  VariableName=T_r_mhe  SampleTime=-1
      settings: Save2DSignal=2-D array (concatenate along first dimension)
  To Workspace5 : ToWorkspace  VariableName=T_w_noisy  SampleTime=-1
      settings: Save2DSignal=2-D array (concatenate along first dimension)
  To Workspace6 : ToWorkspace  VariableName=T_r_noisy  SampleTime=-1
      settings: Save2DSignal=2-D array (concatenate along first dimension)
  To Workspace7 : ToWorkspace  VariableName=T_w  SampleTime=-1
      settings: Save2DSignal=2-D array (concatenate along first dimension)
  To Workspace8 : ToWorkspace  VariableName=T_r  SampleTime=-1
      settings: Save2DSignal=2-D array (concatenate along first dimension)
  s_ref12 : ToWorkspace  VariableName=E_total  SampleTime=-1
      settings: Save2DSignal=2-D array (concatenate along first dimension)
  s_ref15 : ToWorkspace  VariableName=E_rekup  SampleTime=-1
      settings: Save2DSignal=2-D array (concatenate along first dimension)
  s_ref16 : ToWorkspace  VariableName=E_delta  SampleTime=-1
      settings: Save2DSignal=2-D array (concatenate along first dimension)
  wires:
  [T_wr] -> Demux/1
  Clock/1 -> To Workspace13/1, To Workspace11/1
  Energy calculation1/1(E_rekup) -> s_ref15/1
  Energy calculation1/2(E_used) -> s_ref12/1
  Energy calculation1/3(E_delta) -> s_ref16/1
  Rate Transition6/1 -> To Workspace1/1
  Rate Transition1/1 -> To Workspace2/1
  Demux/1 -> Rate Transition6/1, To Workspace7/1
  Demux/2 -> Rate Transition1/1, To Workspace8/1
  [v_ist] -> Rate Transition2/1, To Workspace20/1
  Rate Transition2/1 -> To Workspace/1
  Demux1/1 -> To Workspace3/1
  Demux1/2 -> To Workspace4/1
  [noisy_meas] -> Demux2/1
  Demux2/1 -> To Workspace5/1
  Demux2/2 -> To Workspace6/1
  [MHE_results] -> Selector1/1
  Selector1/1 -> Demux1/1  "MHE"

== system Offline_MiL_Sim_Public/State-Estimation ==
  orig_temp : Inport
  noisy_temp : Inport  Port=2
  LSTM_temp : Inport  Port=3
  Velocity : Inport  Port=4
  Constant2 : Constant  Value=SE_selector_sim
  Multiport Switch : MultiPortSwitch  Inputs=2  SaturateOnIntegerOverflow=off  InputSameDT=off
  Mux4 : Mux  Inputs=2
  Mux7 : Mux  Inputs=2
  Terminator1 : Terminator
  moving_horizon_estimator : Subsystem
  Output : Outport
  wires:
  Velocity/1 -> Mux7/2, Mux4/2, moving_horizon_estimator/2(Velocity)
  noisy_temp/1 -> moving_horizon_estimator/1(noisy_temp)
  orig_temp/1 -> Mux7/1
  LSTM_temp/1 -> Terminator1/1
  moving_horizon_estimator/1(Output) -> Mux4/1
  Mux4/1 -> Multiport Switch/2
  Multiport Switch/1 -> Output/1
  Constant2/1 -> Multiport Switch/1
  Mux7/1 -> Multiport Switch/3

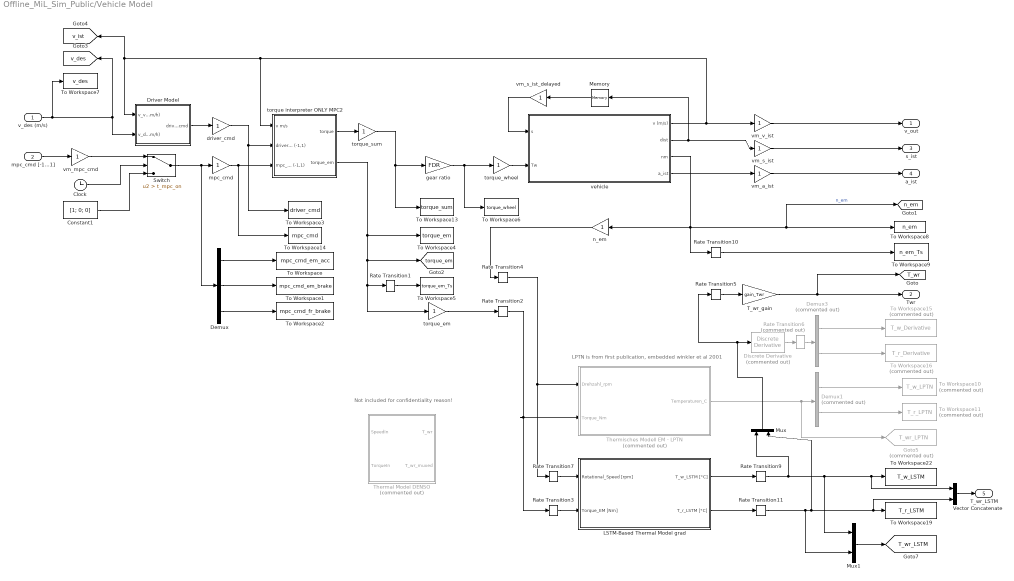
== system Offline_MiL_Sim_Public/Vehicle Model ==
  note: LPTN is from first publication, embedded winkler et al 2001
  note: Not included for confidentiality reason!
  " v_des (m/s)" : Inport  PortDimensions=1
  mpc_cmd [-1...1] : Inport  Port=2  PortDimensions=3
  Clock : Clock
  Constant1 : Constant  Value=[1; 0; 0]
  Demux : Demux  Outputs=3
  Demux1 : Demux  Commented=on  Outputs=2
  Demux3 : Demux  Commented=on  Outputs=2
  Discrete Derivative : simulink/Discrete/Discrete Derivative  Commented=on  gainval=1.0  ICPrevScaledInput=600  OutMin=[]  OutMax=[]  OutDataType=fixdt(1, 16)  OutScaling=2^-10  DoSatur=off
  Driver Model : Subsystem
  Goto5 : Goto  Commented=on  GotoTag=T_wr_LPTN  TagVisibility=global
  LSTM-Based Thermal Model grad : Subsystem
  Memory : Memory  InheritSampleTime=on
  Mux : Mux  Inputs=2
  Mux1 : Mux  Inputs=2
  Rate Transition1 : RateTransition  InitialCondition=n_0  OutPortSampleTime=options.Ts
  Rate Transition10 : RateTransition  InitialCondition=n_0  OutPortSampleTime=options.Ts
  Rate Transition11 : RateTransition  InitialCondition=T_r_0  OutPortSampleTime=step_size
  Rate Transition2 : RateTransition  InitialCondition=M_EM_acc_0  OutPortSampleTime=step_size
  Rate Transition3 : RateTransition  InitialCondition=M_EM_acc_0  OutPortSampleTime=options.Ts
  Rate Transition4 : RateTransition  InitialCondition=n_0  OutPortSampleTime=step_size
  Rate Transition5 : RateTransition  InitialCondition=[T_w_0 T_r_0]  OutPortSampleTime=step_size
  Rate Transition6 : RateTransition  Commented=on  InitialCondition=[0 0]  OutPortSampleTime=step_size
  Rate Transition7 : RateTransition  InitialCondition=n_0  OutPortSampleTime=options.Ts
  Rate Transition9 : RateTransition  InitialCondition=T_w_0  OutPortSampleTime=step_size
  Switch : Switch  Criteria=u2 > Threshold  Threshold=t_mpc_on  SaturateOnIntegerOverflow=off  InputSameDT=off
  T_wr_gain : Gain  Gain=gain_Twr
  Thermal Model DENSO : Subsystem  Commented=on
  Thermisches Modell EM - LPTN : Subsystem  Commented=on
  To Workspace : ToWorkspace  VariableName=mpc_cmd_em_acc  SampleTime=-1
      settings: Save2DSignal=2-D array (concatenate along first dimension)
  To Workspace1 : ToWorkspace  VariableName=mpc_cmd_em_brake  SampleTime=-1
      settings: Save2DSignal=2-D array (concatenate along first dimension)
  To Workspace10 : ToWorkspace  Commented=on  VariableName=T_w_LPTN  SampleTime=-1
      settings: Save2DSignal=2-D array (concatenate along first dimension)
  To Workspace11 : ToWorkspace  Commented=on  VariableName=T_r_LPTN  SampleTime=-1
      settings: Save2DSignal=2-D array (concatenate along first dimension)
  To Workspace13 : ToWorkspace  VariableName=torque_sum  SampleTime=-1
      settings: Save2DSignal=2-D array (concatenate along first dimension)
  To Workspace14 : ToWorkspace  VariableName=mpc_cmd  SampleTime=-1
      settings: Save2DSignal=2-D array (concatenate along first dimension)
  To Workspace15 : ToWorkspace  Commented=on  VariableName=T_w_Derivative  SampleTime=-1
      settings: Save2DSignal=2-D array (concatenate along first dimension)
  To Workspace16 : ToWorkspace  Commented=on  VariableName=T_r_Derivative  SampleTime=-1
      settings: Save2DSignal=2-D array (concatenate along first dimension)
  To Workspace19 : ToWorkspace  VariableName=T_r_LSTM  SampleTime=-1
      settings: Save2DSignal=2-D array (concatenate along first dimension)
  To Workspace2 : ToWorkspace  VariableName=mpc_cmd_fr_brake  SampleTime=-1
      settings: Save2DSignal=2-D array (concatenate along first dimension)
  To Workspace22 : ToWorkspace  VariableName=T_w_LSTM  SampleTime=-1
      settings: Save2DSignal=2-D array (concatenate along first dimension)
  To Workspace3 : ToWorkspace  VariableName=driver_cmd  SampleTime=-1
      settings: Save2DSignal=2-D array (concatenate along first dimension)
  To Workspace4 : ToWorkspace  VariableName=torque_em  SampleTime=-1
      settings: Save2DSignal=2-D array (concatenate along first dimension)
  To Workspace5 : ToWorkspace  VariableName=torque_em_Ts  SampleTime=-1
      settings: Save2DSignal=2-D array (concatenate along first dimension)
  To Workspace6 : ToWorkspace  VariableName=torque_wheel  SampleTime=-1
      settings: Save2DSignal=2-D array (concatenate along first dimension)
  To Workspace7 : ToWorkspace  VariableName=v_des  SampleTime=-1
      settings: Save2DSignal=2-D array (concatenate along first dimension)
  To Workspace8 : ToWorkspace  VariableName=n_em  SampleTime=-1
      settings: Save2DSignal=2-D array (concatenate along first dimension)
  To Workspace9 : ToWorkspace  VariableName=n_em_Ts  SampleTime=-1
      settings: Save2DSignal=2-D array (concatenate along first dimension)
  Vector Concatenate : Concatenate
  driver_cmd : Gain
  gear ratio : Gain  Gain=FDR
  mpc_cmd : Gain
  n_em : Gain
  torque interpreter ONLY MPC2 : Subsystem
  torque_em : Gain
  torque_sum : Gain
  torque_wheel : Gain
  vehicle : Subsystem
  vm_a_ist : Gain
  vm_mpc_cmd : Gain
  vm_s_ist : Gain
  vm_s_ist_delayed : Gain
  vm_v_ist : Gain
  v_out : Outport  SampleTime=step_size  VectorParamsAs1DForOutWhenUnconnected=off
  Twr : Outport  Port=2  PortDimensions=2  VectorParamsAs1DForOutWhenUnconnected=off
  s_ist : Outport  Port=3  SampleTime=step_size  VectorParamsAs1DForOutWhenUnconnected=off
  a_ist : Outport  Port=4  SampleTime=step_size  VectorParamsAs1DForOutWhenUnconnected=off
  T_wr_LSTM : Outport  Port=5
  tag scope: T_wr=global, T_wr_LSTM=global, n_em=global, torque_em=global, v_des=global, v_ist=global
  wires:
  vehicle/1(v (m/s)) -> [v_ist], Driver Model/1(v_veh (km/h)), torque interpreter ONLY MPC2/1(v m/s), vm_v_ist/1
  vehicle/3(nm) -> n_em/1, Rate Transition10/1, [n_em], To Workspace8/1  "n_em"
  " v_des (m/s)"/1 -> Driver Model/2(v_des (km/h)), [v_des], To Workspace7/1
  torque interpreter ONLY MPC2/2(torque_em) -> [torque_em], Rate Transition1/1, torque_em/1, To Workspace4/1
  gear ratio/1 -> torque_wheel/1, To Workspace6/1
  mpc_cmd [-1...1]/1 -> vm_mpc_cmd/1
  Clock/1 -> Switch/2
  Constant1/1 -> Switch/3
  vehicle/2(dist) -> vm_s_ist/1, Memory/1
  Driver Model/1(driver_cmd) -> driver_cmd/1
  driver_cmd/1 -> torque interpreter ONLY MPC2/2(driver_cmd (-1,1)), To Workspace3/1
  torque_em/1 -> Rate Transition2/1
  vm_v_ist/1 -> v_out/1
  vm_s_ist/1 -> s_ist/1
  vm_a_ist/1 -> a_ist/1
  torque_sum/1 -> To Workspace13/1, gear ratio/1
  torque_wheel/1 -> vehicle/2(Tw)
  vm_s_ist_delayed/1 -> vehicle/1(s)
  vm_mpc_cmd/1 -> Switch/1
  n_em/1 -> Rate Transition4/1
  Demux/3 -> To Workspace2/1
  Demux/2 -> To Workspace1/1
  Switch/1 -> Demux/1, mpc_cmd/1
  Demux/1 -> To Workspace/1
  mpc_cmd/1 -> torque interpreter ONLY MPC2/3(mpc_cmd (-1,1)), To Workspace14/1
  Rate Transition1/1 -> To Workspace5/1
  Rate Transition10/1 -> To Workspace9/1
  vehicle/4(a_ist) -> vm_a_ist/1
  Rate Transition4/1 -> Rate Transition7/1, Thermisches Modell EM - LPTN/1(Drehzahl_rpm)
  Rate Transition5/1 -> T_wr_gain/1
  Demux1/2 -> To Workspace11/1
  Demux1/1 -> To Workspace10/1
  Thermisches Modell EM - LPTN/1(Temperaturen_C) -> Goto5/1, Demux1/1
  Memory/1 -> vm_s_ist_delayed/1
  torque interpreter ONLY MPC2/1(torque) -> torque_sum/1
  Rate Transition6/1 -> Demux3/1
  Discrete Derivative/1 -> Rate Transition6/1
  Demux3/1 -> To Workspace15/1
  Demux3/2 -> To Workspace16/1
  Mux1/1 -> [T_wr_LSTM]
  LSTM-Based Thermal Model grad/2(T_r_LSTM [°C]) -> Rate Transition11/1
  LSTM-Based Thermal Model grad/1(T_w_LSTM [°C]) -> Rate Transition9/1
  Rate Transition3/1 -> LSTM-Based Thermal Model grad/2(Torque_EM [Nm])
  Rate Transition7/1 -> LSTM-Based Thermal Model grad/1(Rotational_Speed [rpm])
  T_wr_gain/1 -> [T_wr], Twr/1
  Rate Transition9/1 -> Mux1/1, Vector Concatenate/1, To Workspace22/1, Mux/1
  Rate Transition11/1 -> Mux/2, Vector Concatenate/2, To Workspace19/1, Mux1/2
  Rate Transition2/1 -> Rate Transition3/1, Thermisches Modell EM - LPTN/2(Torque_Nm)
  Vector Concatenate/1 -> T_wr_LSTM/1
  Mux/1 -> Rate Transition5/1, Discrete Derivative/1

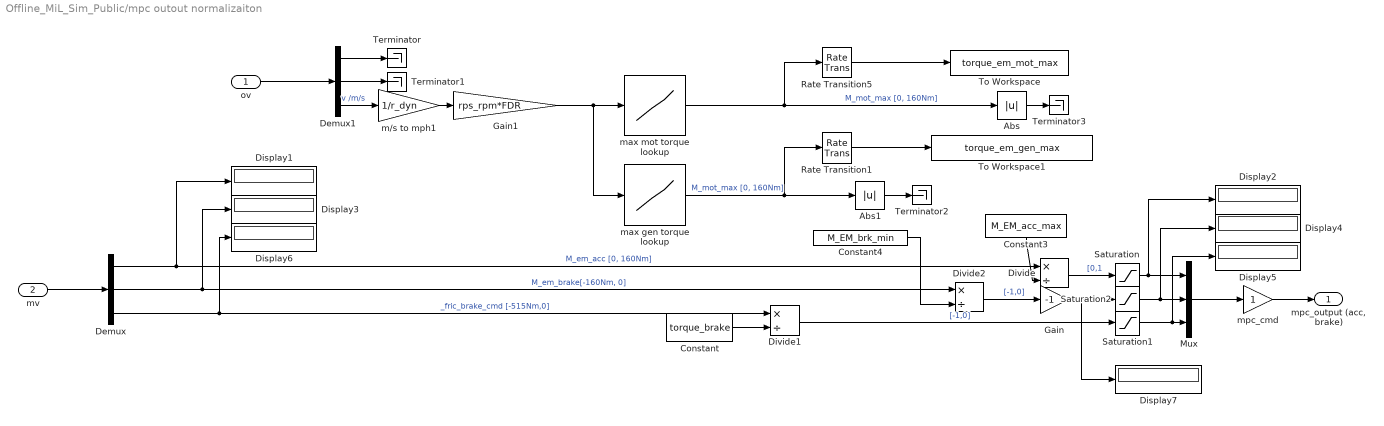
== system Offline_MiL_Sim_Public/mpc outout normalizaiton ==
  ov : Inport  PortDimensions=3
  mv : Inport  Port=2
  Abs : Abs  SaturateOnIntegerOverflow=off
  Abs1 : Abs  SaturateOnIntegerOverflow=off
  Constant : Constant  Value=torque_brake
  Constant3 : Constant  Value=M_EM_acc_max
  Constant4 : Constant  Value=M_EM_brk_min
  Demux : Demux  Outputs=3
  Demux1 : Demux  Outputs=3
  Display{1..7} (7 alike) : Display
  Divide : Product  Inputs=*/
  Divide1 : Product  Inputs=*/
  Divide2 : Product  Inputs=*/
  Gain : Gain  Gain=-1
  Gain1 : Gain  Gain=rps_rpm*FDR
  Mux : Mux  Inputs=3
  Rate Transition1 : RateTransition  OutPortSampleTime=step_size
  Rate Transition5 : RateTransition  OutPortSampleTime=step_size
  Saturation : Saturate  UpperLimit=1  LowerLimit=0
  Saturation1 : Saturate  UpperLimit=0  LowerLimit=-1
  Saturation2 : Saturate  UpperLimit=0  LowerLimit=-1
  Terminator{,1..3} (4 alike) : Terminator
  To Workspace : ToWorkspace  VariableName=torque_em_mot_max  SampleTime=-1
      settings: Save2DSignal=2-D array (concatenate along first dimension)
  To Workspace1 : ToWorkspace  VariableName=torque_em_gen_max  SampleTime=-1
      settings: Save2DSignal=2-D array (concatenate along first dimension)
  m/s to mph1 : Gain  Gain=1/r_dyn  SaturateOnIntegerOverflow=on  OutDataTypeStr=Inherit: Same as input  ParamDataTypeStr=Inherit: Same as input
  max gen torque lookup : Lookup_n-D  NumberOfTableDimensions=1  BreakpointsForDimension1=n_gen_max  Table=M_gen_max  InternalRulePriority=Speed  RndMeth=Simplest
  max mot torque lookup : Lookup_n-D  NumberOfTableDimensions=1  BreakpointsForDimension1=n_mot_max  Table=M_mot_max  InternalRulePriority=Speed  RndMeth=Simplest
  mpc_cmd : Gain
  "mpc_output (acc, brake)" : Outport  VectorParamsAs1DForOutWhenUnconnected=off
  wires:
  Gain1/1 -> max gen torque lookup/1, max mot torque lookup/1
  Divide/1 -> Saturation/1  "[0,1"
  m/s to mph1/1 -> Gain1/1
  ov/1 -> Demux1/1
  Constant/1 -> Divide1/2
  Divide2/1 -> Gain/1  "[-1,0]"
  Saturation/1 -> Mux/1, Display2/1
  Saturation1/1 -> Display5/1, Mux/3
  Saturation2/1 -> Mux/2, Display4/1
  Mux/1 -> mpc_cmd/1
  Demux1/3 -> m/s to mph1/1  "v /m/s"
  Demux1/1 -> Terminator/1
  Demux1/2 -> Terminator1/1
  mpc_cmd/1 -> "mpc_output (acc, brake)"/1
  Rate Transition5/1 -> To Workspace/1
  max mot torque lookup/1 -> Abs/1, Rate Transition5/1  "M_mot_max [0, 160Nm]"
  max gen torque lookup/1 -> Rate Transition1/1, Abs1/1  "M_mot_max [0, 160Nm]"
  Rate Transition1/1 -> To Workspace1/1
  Abs1/1 -> Terminator2/1
  Abs/1 -> Terminator3/1
  Constant3/1 -> Divide/2
  Constant4/1 -> Divide2/2
  Divide1/1 -> Saturation1/1  "[-1,0]"
  mv/1 -> Demux/1
  Gain/1 -> Display7/1, Saturation2/1
  Demux/3 -> Divide1/1, Display6/1  "_fric_brake_cmd [-515Nm,0]"
  Demux/2 -> Divide2/1, Display3/1  "M_em_brake[-160Nm, 0]"
  Demux/1 -> Display1/1, Divide/1  "M_em_acc [0, 160Nm]"

== system Offline_MiL_Sim_Public/uminmax ==
  v_preview (m/s) : Inport
  Gain1 : Gain  Gain=rps_rpm*FDR
  "M_em,acc, max" : Constant  Value=0
  "M_em,acc, min" : Constant  Value=0
  M_frict _brake max : Constant  Value=0
  M_frict _brake min : Constant  Value=-torque_brake
  Matrix Concatenate : Concatenate  NumInputs=3  Mode=Multidimensional array  ConcatenateDimension=2
  Matrix Concatenate1 : Concatenate  NumInputs=3  Mode=Multidimensional array  ConcatenateDimension=2
  Product{,1..3} (4 alike) : Product
  horizon1 : Constant  Value=ones(options.P,1)
  horizon2 : Constant  Value=ones(options.P,1)
  m/s to mph1 : Gain  Gain=1/r_dyn  SaturateOnIntegerOverflow=on  OutDataTypeStr=Inherit: Same as input  ParamDataTypeStr=Inherit: Same as input
  max gen torque lookup : Lookup_n-D  NumberOfTableDimensions=1  BreakpointsForDimension1=n_gen_max  Table=M_gen_max  InternalRulePriority=Speed  RndMeth=Simplest
  max mot torque lookup : Lookup_n-D  NumberOfTableDimensions=1  BreakpointsForDimension1=n_mot_max  Table=M_mot_max  InternalRulePriority=Speed  RndMeth=Simplest
  umin : Outport  VectorParamsAs1DForOutWhenUnconnected=off
  umax : Outport  Port=2  VectorParamsAs1DForOutWhenUnconnected=off
  wires:
  Gain1/1 -> max gen torque lookup/1, max mot torque lookup/1
  m/s to mph1/1 -> Gain1/1
  v_preview (m/s)/1 -> m/s to mph1/1
  horizon1/1 -> Product1/1, Product/1
  "M_em,acc, max"/1 -> Product/2
  M_frict _brake max/1 -> Product1/2
  "M_em,acc, min"/1 -> Product2/2
  horizon2/1 -> Product3/1, Product2/1
  M_frict _brake min/1 -> Product3/2
  Product/1 -> Matrix Concatenate/2
  Matrix Concatenate1/1 -> umin/1
  max gen torque lookup/1 -> Matrix Concatenate1/2
  Product2/1 -> Matrix Concatenate1/1
  Product3/1 -> Matrix Concatenate1/3
  Product1/1 -> Matrix Concatenate/3
  max mot torque lookup/1 -> Matrix Concatenate/1
  Matrix Concatenate/1 -> umax/1

== system Offline_MiL_Sim_Public/Distance Check/Distance Change Security Check ==
  s : Inport
  Constant : Constant  Value=start_distance_check
  Constant1 : Constant  Value=break_criteria
  MATLAB Function : MATLAB Function  TreatAsAtomicUnit=on
  Memory : Memory  InheritSampleTime=on
  bool_stop : Outport
  wires:
  Memory/1 -> MATLAB Function/2(s_old)
  s/1 -> Memory/1, MATLAB Function/1(s)
  MATLAB Function/1(bool_stop) -> bool_stop/1
  Constant1/1 -> MATLAB Function/4(break_criteria)
  Constant/1 -> MATLAB Function/3(start_distance_check)

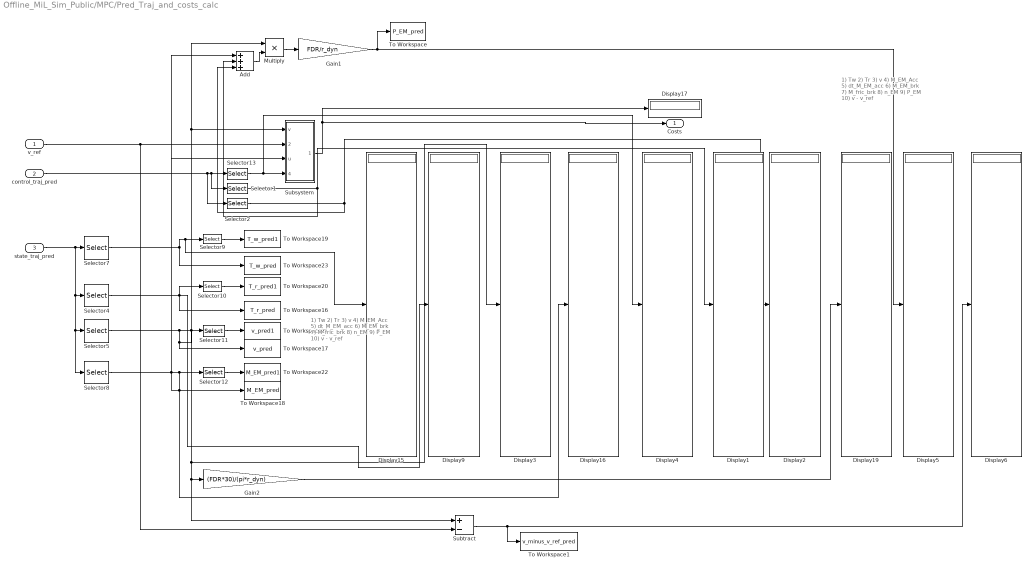
== system Offline_MiL_Sim_Public/MPC/Pred_Traj_and_costs_calc ==
  note: 1) Tw
      | 2) Tr
      | 3) v
      | 4) M_EM_Acc
      | 5) dt_M_EM_acc
      | 6) M_EM_brk
      | 7) M_fric_brk
      | 8) n_EM
      | 9) P_EM
      | 10) v - v_ref
  note: 1) Tw
      | 2) Tr
      | 3) v
      | 4) M_EM_Acc
      | 5) dt_M_EM_acc
      | 6) M_EM_brk
      | 7) M_fric_brk
      | 8) n_EM
      | 9) P_EM
      | 10) v - v_ref
  v_ref : Inport
  control_traj_pred : Inport  Port=2
  state_traj_pred : Inport  Port=3
  Add : Sum  Inputs=+++
  Display{1..6,9,15..17,19} (11 alike) : Display
  Gain1 : Gain  Gain=FDR/r_dyn
  Gain2 : Gain  Gain=(FDR*30)/(pi*r_dyn)
  Multiply : Product
  Selector1 : Selector  InputPortWidth=options.n_controls*options.P  IndexOptions=Index vector (dialog)  Indices=[2:options.n_controls:options.n_controls*options.P]  OutputSizes=1
  Selector{9..12} (4 alike) : Selector  InputPortWidth=options.P  IndexOptions=Index vector (dialog)  Indices=[1]  OutputSizes=1
  Selector13 : Selector  InputPortWidth=options.n_controls*options.P  IndexOptions=Index vector (dialog)  Indices=[1:options.n_controls:options.n_controls*options.P]  OutputSizes=1
  Selector2 : Selector  InputPortWidth=options.n_controls*options.P  IndexOptions=Index vector (dialog)  Indices=[3:options.n_controls:options.n_controls*options.P]  OutputSizes=1
  Selector4 : Selector  InputPortWidth=options.n_states*options.P  IndexOptions=Index vector (dialog)  Indices=[2:options.n_states:options.n_states*options.P-2]  OutputSizes=1
  Selector5 : Selector  InputPortWidth=options.n_states*options.P  IndexOptions=Index vector (dialog)  Indices=[3:options.n_states:options.n_states*options.P-1]  OutputSizes=1
  Selector7 : Selector  InputPortWidth=options.n_states*options.P  IndexOptions=Index vector (dialog)  Indices=[1:options.n_states:options.n_states*options.P-3]  OutputSizes=1
  Selector8 : Selector  InputPortWidth=options.n_states*options.P  IndexOptions=Index vector (dialog)  Indices=[options.n_states:options.n_states:options.n_states*options.P]  OutputSizes=1
  Subsystem : Subsystem
  Subtract : Sum  Inputs=+-
  To Workspace : ToWorkspace  VariableName=P_EM_pred  SaveFormat=Timeseries  SampleTime=-1
  To Workspace1 : ToWorkspace  VariableName=v_minus_v_ref_pred  SaveFormat=Timeseries  SampleTime=-1
  To Workspace16 : ToWorkspace  VariableName=T_r_pred  SampleTime=-1
  To Workspace17 : ToWorkspace  VariableName=v_pred  SampleTime=-1
  To Workspace18 : ToWorkspace  VariableName=M_EM_pred  SampleTime=-1
  To Workspace19 : ToWorkspace  VariableName=T_w_pred1  SampleTime=-1
  To Workspace20 : ToWorkspace  VariableName=T_r_pred1  SampleTime=-1
  To Workspace21 : ToWorkspace  VariableName=v_pred1  SampleTime=-1
  To Workspace22 : ToWorkspace  VariableName=M_EM_pred1  SampleTime=-1
  To Workspace23 : ToWorkspace  VariableName=T_w_pred  SampleTime=-1
  Costs : Outport  VectorParamsAs1DForOutWhenUnconnected=off
  wires:
  Selector7/1 -> Selector9/1, Display15/1, To Workspace23/1
  state_traj_pred/1 -> Selector8/1, Selector5/1, Selector4/1, Selector7/1
  Selector10/1 -> To Workspace20/1
  Selector8/1 -> Add/1, Display16/1, To Workspace18/1, Selector12/1, Subsystem/3(u)
  Selector5/1 -> Subtract/1, Gain2/1, Display3/1, Selector11/1, Multiply/1, Subsystem/1(v), To Workspace17/1
  v_ref/1 -> Subtract/2, Subsystem/2(v_ref)
  Selector9/1 -> To Workspace19/1
  Selector4/1 -> To Workspace16/1, Selector10/1, Display9/1
  control_traj_pred/1 -> Selector2/1, Selector1/1, Selector13/1
  Selector13/1 -> Display4/1, Subsystem/4(dt_u)
  Subsystem/1(cost) -> Display17/1, Costs/1
  Selector11/1 -> To Workspace21/1
  Selector12/1 -> To Workspace22/1
  Gain2/1 -> Display19/1
  Selector1/1 -> Display1/1, Add/2
  Selector2/1 -> Display2/1, Add/3
  Multiply/1 -> Gain1/1
  Gain1/1 -> Display5/1, To Workspace/1
  Add/1 -> Multiply/2
  Subtract/1 -> Display6/1, To Workspace1/1

== system Offline_MiL_Sim_Public/MPC/SolverStop ==
  solver_status : Inport
  Clock : Clock
  Constant : Constant  Value=0
  MATLAB Function : MATLAB Function  TreatAsAtomicUnit=on
  Switch : Switch  Criteria=u2 > Threshold  Threshold=t_mpc_on  SaturateOnIntegerOverflow=off  InputSameDT=off
  bool_stop : Outport
  wires:
  MATLAB Function/1(bool_stop) -> bool_stop/1
  Clock/1 -> Switch/2
  Constant/1 -> Switch/3
  solver_status/1 -> Switch/1
  Switch/1 -> MATLAB Function/1(solver_status)
